simulink model "lab_04_simulink"  (R2024b)
settings: Solver=VariableStepAuto  StartTime=0.0  StopTime=10.0  RelTol=1e-3
settings RTWCC: GenCodeOnly=on

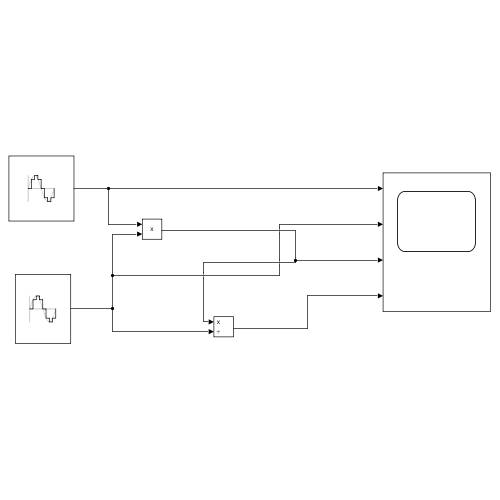
[thumbnail: Simulink's stored preview of the top-level diagram]
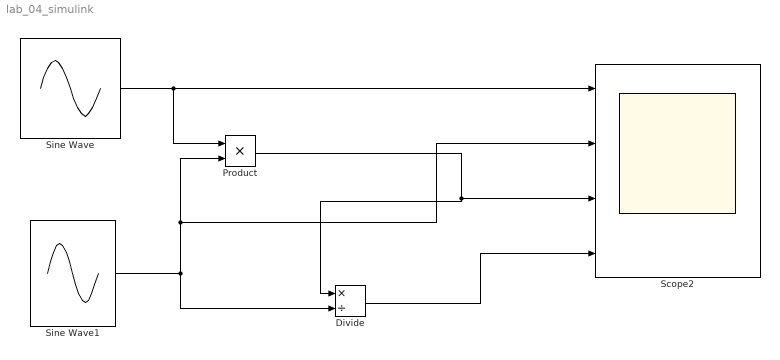
== system lab_04_simulink ==
  Divide : Product  Inputs=*/
  Product : Product
  Scope2 : Scope  NumInputPorts=4
  Sine Wave : Sin  Amplitude=2  SampleTime=0.01
  Sine Wave1 : Sin  Amplitude=2  Frequency=10  SampleTime=0.01
  wires:
  Sine Wave/1 -> Scope2/1, Product/1
  Sine Wave1/1 -> Divide/2, Scope2/2, Product/2
  Product/1 -> Divide/1, Scope2/3
  Divide/1 -> Scope2/4
